simulink model "model1"  (R2018b)
settings: Solver=VariableStepAuto  StartTime=0.0  StopTime=300  RelTol=1e-3
values from neighbouring files (symbols this model uses):
  SP = 0.5    [e1.m]
  T = 45    [e1.m]
  tau = 22    [e1.m]
undefined symbols (not defined in the file or in its folder): h
settings Model: Creator=podstawy  LastModifiedBy=podstawy

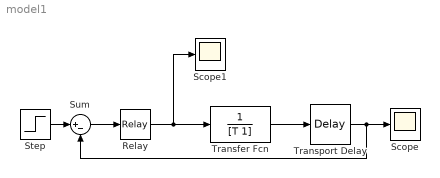
== system model1 ==
  Relay : Relay  OnSwitchValue=h  OffSwitchValue=-h
  Scope : Scope
  Scope1 : Scope
  Step : Step  After=SP  SampleTime=0
  Sum : Sum  Inputs=|+-
  Transfer Fcn : TransferFcn  Denominator=[T 1]
  Transport Delay : TransportDelay  DelayTime=tau
  wires:
  Step/1 -> Sum/1
  Sum/1 -> Relay/1
  Relay/1 -> Transfer Fcn/1, Scope1/1
  Transfer Fcn/1 -> Transport Delay/1
  Transport Delay/1 -> Sum/2, Scope/1
